simulink library "HEV_Animation_Lib"  (R2015b)
settings: Solver=ode45  StartTime=0.0  StopTime=10.0  RelTol=1e-3
Description:
  | Copyright 2014-2015 The MathWorks, Inc.
settings Model: Creator=smiller  LastModifiedBy=smiller
settings DataIOCC: SaveFormat=Array  SignalLoggingSaveFormat=ModelDataLogs
settings OptimizationCC: ExpressionDepthLimit=2147483647
settings DebuggingCC: UnderspecifiedInitializationDetection=Classic  MergeDetectMultiDrivingBlocksExec=none  SolverPrmCheckMsg=warning  FcnCallInpInsideContextMsg=UseLocalSettings  StateNameClashWarn=warning
settings HardwareCC: ProdBitPerPointer=32  ProdLargestAtomicFloat=None  ProdIntDivRoundTo=Undefined  ProdEndianess=Unspecified  ProdWordSize=32  ProdHWDeviceType=32-bit Generic
settings GRTTargetCC: GeneratePreprocessorConditionals=Disable all  CombineOutputUpdateFcns=off  GRTInterface=on
settings ConfigComp: CovModelRefEnable=Off  CovSFcnEnable=off

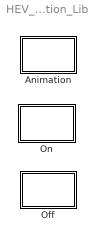
== system HEV_Animation_Lib ==
  Animation : Subsystem  BlockChoice=Off
      mask init:
      | Configure_HEV_Animation
      settings: TemplateBlock=self  MemberBlocks=Off,On
  Off : Subsystem
      mask Display:
      | color('gray');
      | disp('Anim.\nOff');
  On : Subsystem
      settings: CopyFcn=|
      | hcar = hybridCar('HEV_SeriesParallel');
      | set(hcar,'position',[7.0000    2.4615  188.6000   46.5385])
      settings: OpenFcn=|
      | hcar = hybridCar('HEV_SeriesParallel');
      | set(hcar,'position',[7.0000    2.4615  188.6000   46.5385])
      mask Display: image(imread('HEV_Sys_GUI.jpg'))

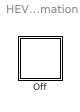
== system HEV_Animation_Lib/Animation ==
  Off : Subsystem

== system HEV_Animation_Lib/Off ==

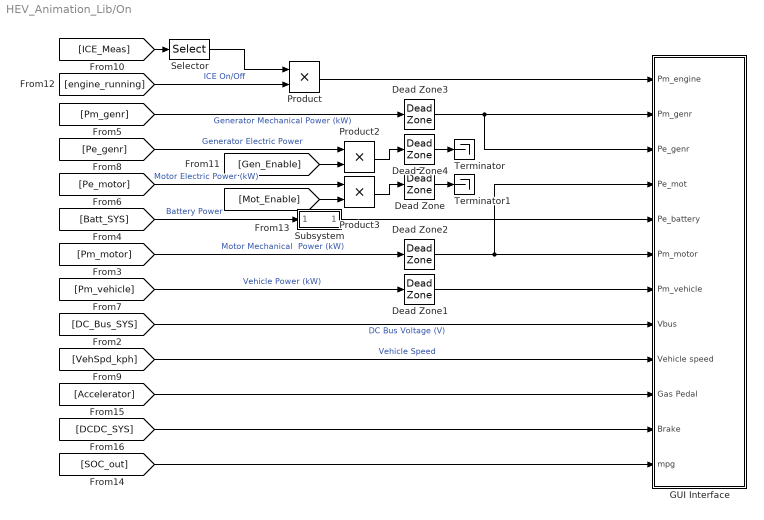
== system HEV_Animation_Lib/On ==
  Dead Zone{,1..4} (5 alike) : DeadZone  LowerValue=-0.1  UpperValue=0.1  SaturateOnIntegerOverflow=on
  GUI Interface : Subsystem
  Product : Product  RndMeth=Zero
  Product2 : Product  RndMeth=Zero
  Product3 : Product  RndMeth=Zero
  Selector : Selector  InputPortWidth=3  IndexOptions=Index vector (dialog)  Indices=[3]  OutputSizes=1
  Subsystem : Subsystem
  Terminator : Terminator
  Terminator1 : Terminator
  wires:
  Selector/1 -> Product/1
  [ICE_Meas] -> Selector/1
  Dead Zone3/1 -> GUI Interface/3(Pe_genr), GUI Interface/2(Pm_genr)
  [SOC_out] -> GUI Interface/12(mpg)
  [Pm_motor] -> Dead Zone2/1  "Motor Mechanical  Power (kW)"
  [Batt_SYS] -> Subsystem/1(In1)  "Battery Power"
  Dead Zone2/1 -> GUI Interface/4(Pe_mot), GUI Interface/6(Pm_motor)
  Dead Zone1/1 -> GUI Interface/7(Pm_vehicle)
  Product3/1 -> Dead Zone/1
  [Mot_Enable] -> Product3/2
  Product2/1 -> Dead Zone4/1
  [Gen_Enable] -> Product2/2
  [engine_running] -> Product/2  "ICE On/Off"
  [Pm_genr] -> Dead Zone3/1  "Generator Mechanical Power (kW)"
  [VehSpd_kph] -> GUI Interface/9(Vehicle speed)  "Vehicle Speed"
  [Pm_vehicle] -> Dead Zone1/1  "Vehicle Power (kW)"
  [DC_Bus_SYS] -> GUI Interface/8(Vbus)  "DC Bus Voltage (V)"
  [Pe_motor] -> Product3/1  "Motor Electric Power (kW)"
  [Pe_genr] -> Product2/1  "Generator Electric Power"
  Subsystem/1(Out1) -> GUI Interface/5(Pe_battery)
  [Accelerator] -> GUI Interface/10(Gas Pedal)
  [DCDC_SYS] -> GUI Interface/11(Brake)
  Product/1 -> GUI Interface/1(Pm_engine)
  Dead Zone4/1 -> Terminator/1
  Dead Zone/1 -> Terminator1/1

== system HEV_Animation_Lib/Animation/Off ==

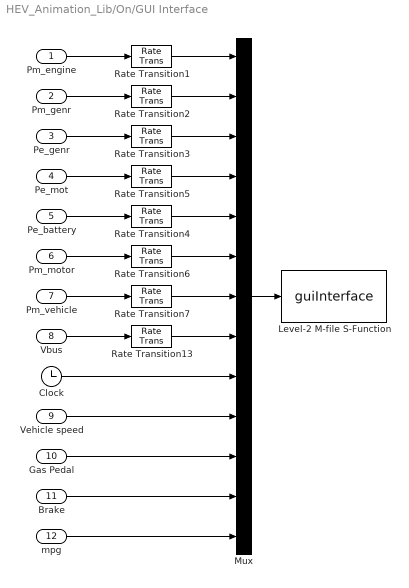
== system HEV_Animation_Lib/On/GUI Interface ==
  Pm_engine : Inport
  Pm_genr : Inport  Port=2
  Pe_genr : Inport  Port=3
  Pe_mot : Inport  Port=4
  Pe_battery : Inport  Port=5
  Pm_motor : Inport  Port=6
  Pm_vehicle : Inport  Port=7
  Vbus : Inport  Port=8
  Vehicle speed : Inport  Port=9
  Gas Pedal : Inport  Port=10
  Brake : Inport  Port=11
  mpg : Inport  Port=12
  Clock : Clock
  Level-2 M-file S-Function : M-S-Function  FunctionName=guiInterface
  Mux : Mux  Inputs=13
  Rate Transition{1..5} (5 alike) : RateTransition  Deterministic=off
  Rate Transition13 : RateTransition  Deterministic=off  OutPortSampleTime=1
  Rate Transition6 : RateTransition  Deterministic=off  OutPortSampleTime=1
  Rate Transition7 : RateTransition  Deterministic=off  OutPortSampleTime=1
  wires:
  Pm_motor/1 -> Rate Transition6/1
  Pm_vehicle/1 -> Rate Transition7/1
  Pe_genr/1 -> Rate Transition3/1
  Pe_battery/1 -> Rate Transition4/1
  Mux/1 -> Level-2 M-file S-Function/1
  Rate Transition2/1 -> Mux/2
  Rate Transition3/1 -> Mux/3
  Rate Transition1/1 -> Mux/1
  Vbus/1 -> Rate Transition13/1
  Pm_genr/1 -> Rate Transition2/1
  Pm_engine/1 -> Rate Transition1/1
  Pe_mot/1 -> Rate Transition5/1
  Rate Transition5/1 -> Mux/4
  Rate Transition4/1 -> Mux/5
  Rate Transition7/1 -> Mux/7
  Rate Transition13/1 -> Mux/8
  Clock/1 -> Mux/9
  Vehicle speed/1 -> Mux/10
  Rate Transition6/1 -> Mux/6
  Gas Pedal/1 -> Mux/11
  Brake/1 -> Mux/12
  mpg/1 -> Mux/13

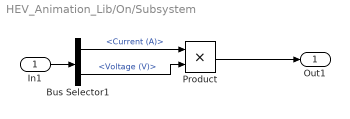
== system HEV_Animation_Lib/On/Subsystem ==
  In1 : Inport
  Bus Selector1 : BusSelector  OutputSignals=Current (A),Voltage (V)
  Product : Product  RndMeth=Zero
  Out1 : Outport
  wires:
  Product/1 -> Out1/1
  Bus Selector1/2 -> Product/2  "<Voltage (V)>"
  In1/1 -> Bus Selector1/1
  Bus Selector1/1 -> Product/1  "<Current (A)>"
